simulink model "pendulumOnACart_disturbance_rejection"  (R2013b)
settings: Solver=ode45  StartTime=0.0  StopTime=20  RelTol=1e-3
InitFcn:
  | pendulumOnACart_disturbance_rejection_init;
values from neighbouring files (symbols this model uses):
  A = [0                      0                           1	0   0 ... (first row only)    [pendulumOnACart_observer_PID_init.m]
  B = [0 ... (first row only)    [pendulumOnACart_observer_PID_init.m]
  C = [0  1  0  0]    [pendulumOnACart_init.m]    (also in pendulumOnACart_observer_PID_init.m = [1  0  0  0  0)
  cM = 5    [pendulumOnACart_init.m]    (also in pendulumOnACart_observer_PID_init.m)
  dt = 1/1000    (= 0.001)    [pendulumOnACart_init.m]    (also in pendulumOnACart_observer_PID_init.m)
  dTheta_init = 2.0    (= 2)    [pendulumOnACart_init.m]    (also in pendulumOnACart_observer_PID_init.m)
  encRez = 12    [pendulumOnACart_init.m]    (also in pendulumOnACart_observer_PID_init.m)
  g = 9.81    [pendulumOnACart_init.m]    (also in pendulumOnACart_observer_PID_init.m)
  K = place(A,B,[p1 p2 p3 p4 p5])    [pendulumOnACart_observer_PID_init.m]
  L = (place(A',C',[p1 p2 p3 p4 p5]))'    [pendulumOnACart_observer_PID_init.m]
  pL = 0.25    [pendulumOnACart_init.m]    (also in pendulumOnACart_observer_PID_init.m)
  pm = 1    [pendulumOnACart_init.m]    (also in pendulumOnACart_observer_PID_init.m)
  theta_init = 0.2    [pendulumOnACart_init.m]    (also in pendulumOnACart_observer_PID_init.m)
undefined symbols (not defined in the file or in its folder): Ka
settings Model: Creator=jaustin  LastModifiedBy=jaustin

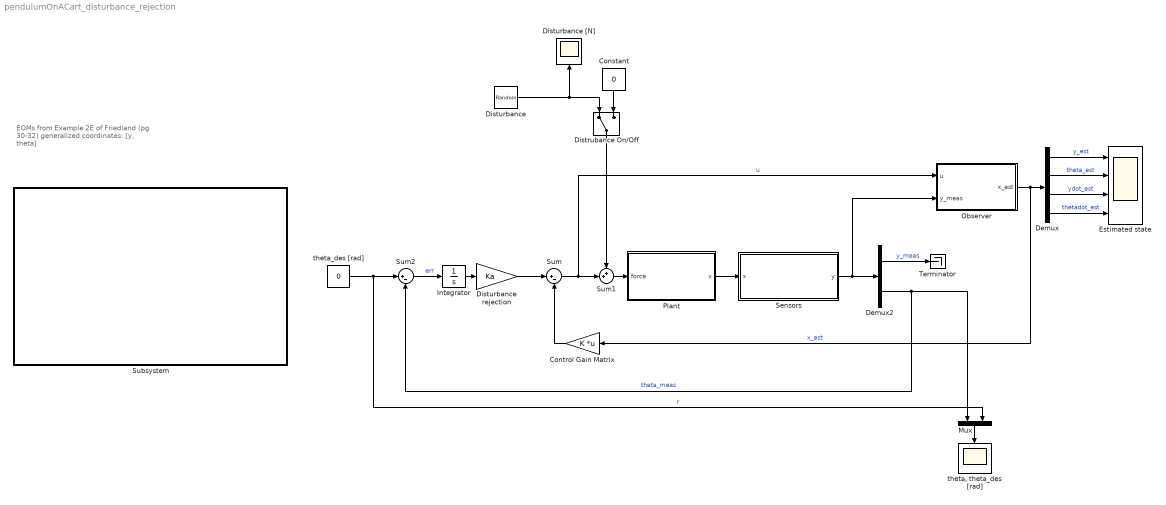
== system pendulumOnACart_disturbance_rejection ==
  note: EOMs from Example 2E of Friedland
      | (pg 30-32)
      |
      | generalized coordinates: [y, theta]
  Constant : Constant  Value=0
  Control Gain Matrix : Gain  Gain=K  Multiplication=Matrix(K*u)
  Demux : Demux
  Demux2 : Demux  Outputs=2
  Distrubance On/Off : ManualSwitch
  Disturbance : RandomNumber  Variance=.5  SampleTime=dt*100
  Disturbance rejection : Gain  Gain=Ka
  Disturbance [N] : Scope
      settings: TimeRange=5  YMin=-20  YMax=80  SaveName=ScopeData7
  Estimated state : Scope  NumInputPorts=4
      settings: TimeRange=20  YMin=0~-1~-6~-2  YMax=10~1~8~1.5  SaveName=ScopeData5
  Integrator : Integrator
  Mux : Mux  Inputs=2
  Observer : Subsystem
  Plant : Subsystem
  Sensors : Subsystem
  Subsystem : Subsystem
      mask Display: image('pendulum_diagram.png')
  Sum : Sum  Inputs=|+-
  Sum1 : Sum  Inputs=++|
  Sum2 : Sum  Inputs=|+-
  Terminator : Terminator
  "theta, theta_des [rad]" : Scope
      settings: TimeRange=20  YMin=-1  YMax=0.8
  theta_des [rad] : Constant  Value=0
  wires:
  Mux/1 -> "theta, theta_des [rad]"/1
  Plant/1(x) -> Sensors/1(x)
  Observer/1(x_est) -> Control Gain Matrix/1, Demux/1  "x_est"
  Sensors/1(y) -> Observer/2(y_meas), Demux2/1
  Demux/1 -> Estimated state/1  "y_est"
  Demux/2 -> Estimated state/2  "theta_est"
  Demux/3 -> Estimated state/3  "ydot_est"
  Demux/4 -> Estimated state/4  "thetadot_est"
  Demux2/2 -> Sum2/2, Mux/1  "theta_meas"
  Sum1/1 -> Plant/1(force)
  Disturbance/1 -> Distrubance On/Off/1, Disturbance [N]/1
  Distrubance On/Off/1 -> Sum1/1
  Constant/1 -> Distrubance On/Off/2
  Demux2/1 -> Terminator/1  "y_meas"
  Sum/1 -> Observer/1(u), Sum1/2  "u"
  Control Gain Matrix/1 -> Sum/2
  theta_des [rad]/1 -> Mux/2, Sum2/1  "r"
  Sum2/1 -> Integrator/1  "err"
  Disturbance rejection/1 -> Sum/1
  Integrator/1 -> Disturbance rejection/1

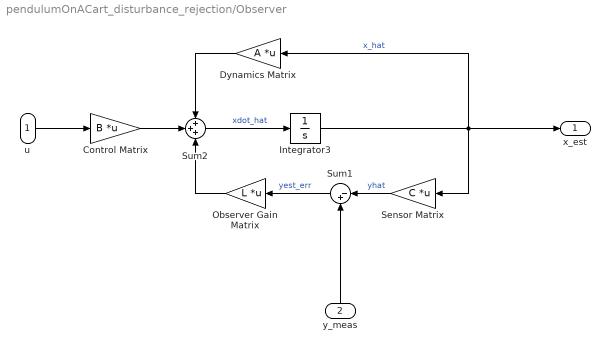
== system pendulumOnACart_disturbance_rejection/Observer ==
  u : Inport
  y_meas : Inport  Port=2
  Control Matrix : Gain  Gain=B  Multiplication=Matrix(K*u)
  Dynamics Matrix : Gain  Gain=A  Multiplication=Matrix(K*u)
  Integrator3 : Integrator
  Observer Gain Matrix : Gain  Gain=L  Multiplication=Matrix(K*u)
  Sensor Matrix : Gain  Gain=C  Multiplication=Matrix(K*u)
  Sum1 : Sum  Inputs=|-+
  Sum2 : Sum  Inputs=+++
  x_est : Outport
  wires:
  Control Matrix/1 -> Sum2/2
  Sum1/1 -> Observer Gain Matrix/1  "yest_err"
  Observer Gain Matrix/1 -> Sum2/3
  Integrator3/1 -> x_est/1, Dynamics Matrix/1, Sensor Matrix/1  "x_hat"
  Dynamics Matrix/1 -> Sum2/1
  Sensor Matrix/1 -> Sum1/1  "yhat"
  Sum2/1 -> Integrator3/1  "xdot_hat"
  y_meas/1 -> Sum1/2
  u/1 -> Control Matrix/1

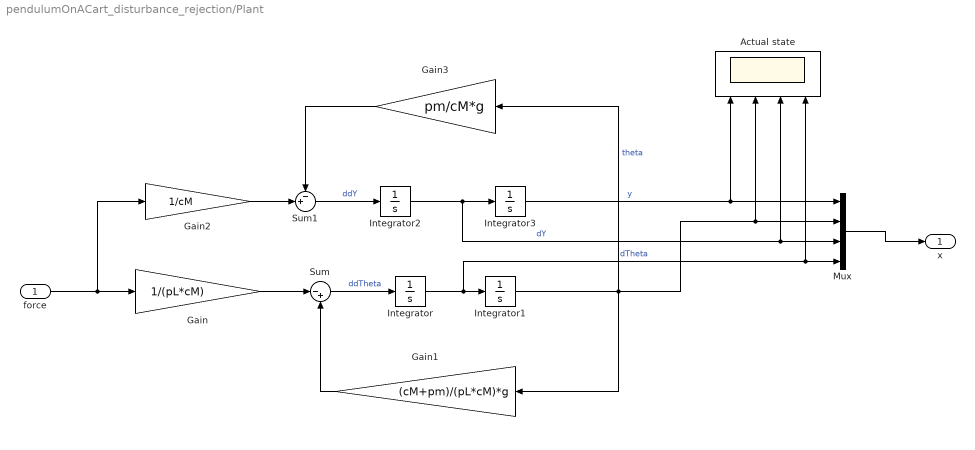
== system pendulumOnACart_disturbance_rejection/Plant ==
  force : Inport
  Actual state : Scope  NumInputPorts=4
      settings: TimeRange=20  YMin=-2~-1~-6~-2  YMax=10~1~8~3  SaveName=ScopeData6
  Gain : Gain  Gain=1/(pL*cM)
  Gain1 : Gain  Gain=(cM+pm)/(pL*cM)*g
  Gain2 : Gain  Gain=1/cM
  Gain3 : Gain  Gain=pm/cM*g
  Integrator : Integrator  InitialCondition=dTheta_init
  Integrator1 : Integrator  InitialCondition=theta_init
  Integrator2 : Integrator
  Integrator3 : Integrator
  Mux : Mux
  Sum : Sum  Inputs=|-+
  Sum1 : Sum  Inputs=-+|
  x : Outport
  wires:
  Integrator1/1 -> Gain3/1, Actual state/2, Mux/2, Gain1/1  "theta"
  Gain2/1 -> Sum1/2
  Sum1/1 -> Integrator2/1  "ddY"
  Integrator2/1 -> Actual state/3, Mux/3, Integrator3/1  "dY"
  Gain/1 -> Sum/1
  force/1 -> Gain2/1, Gain/1
  Gain1/1 -> Sum/2
  Gain3/1 -> Sum1/1
  Integrator/1 -> Actual state/4, Mux/4, Integrator1/1  "dTheta"
  Sum/1 -> Integrator/1  "ddTheta"
  Mux/1 -> x/1
  Integrator3/1 -> Actual state/1, Mux/1  "y"

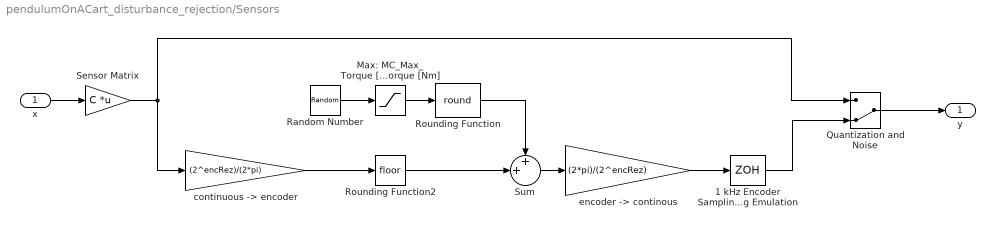
== system pendulumOnACart_disturbance_rejection/Sensors ==
  x : Inport
  1 kHz Encoder Sampling Emulation : ZeroOrderHold  SampleTime=dt
  Max: MC_Max_Torque [Nm] Min: MC_Min_Torque [Nm] : Saturate  UpperLimit=1  LowerLimit=-1
  Quantization and Noise : ManualSwitch  CurrentSetting=0
  Random Number : RandomNumber  Variance=0.5  SampleTime=dt*10
  Rounding Function : Rounding  Operator=round
  Rounding Function2 : Rounding
  Sensor Matrix : Gain  Gain=C  Multiplication=Matrix(K*u)
  Sum : Sum  Inputs=++|
  "continuous -> encoder" : Gain  Gain=(2^encRez)/(2*pi)
  "encoder -> continous" : Gain  Gain=(2*pi)/(2^encRez)
  y : Outport
  wires:
  Quantization and Noise/1 -> y/1
  x/1 -> Sensor Matrix/1
  "continuous -> encoder"/1 -> Rounding Function2/1
  Rounding Function2/1 -> Sum/2
  Random Number/1 -> Max: MC_Max_Torque [Nm] Min: MC_Min_Torque [Nm]/1
  Max: MC_Max_Torque [Nm] Min: MC_Min_Torque [Nm]/1 -> Rounding Function/1
  Sum/1 -> "encoder -> continous"/1
  Rounding Function/1 -> Sum/1
  "encoder -> continous"/1 -> 1 kHz Encoder Sampling Emulation/1
  1 kHz Encoder Sampling Emulation/1 -> Quantization and Noise/2
  Sensor Matrix/1 -> Quantization and Noise/1, "continuous -> encoder"/1

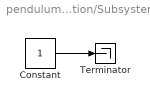
== system pendulumOnACart_disturbance_rejection/Subsystem ==
  Constant : Constant
  Terminator : Terminator
  wires:
  Constant/1 -> Terminator/1
